simulink model "dc_motor_sim_model"  (R2017a)
settings: Solver=FixedStepAuto  StartTime=0.0  StopTime=0.5  FixedStep=1e-4  RelTol=1e-3
InitFcn:
  | Tw=0.01;     %Ancho de Ventana.
  | ppv=20;      %Pulsos por vuelta.
  | Ts=1e-4;     %Tiempo de muestreo.
  | 
  | num=[0 0.7770 0];
  | den=[1.0000 -0.9918 -0.0061];
settings Model: Creator=Martin  LastModifiedBy=Martin

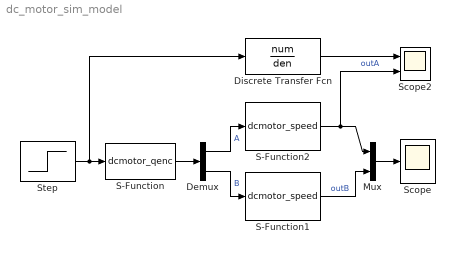
== system dc_motor_sim_model ==
  Demux : Demux  Outputs=2
  Discrete Transfer Fcn : DiscreteTransferFcn  Numerator=num  Denominator=den  SampleTime=Ts
  Mux : Mux  Inputs=2
  S-Function : S-Function  FunctionName=dcmotor_qenc  Parameters=ppv  SFunctionDeploymentMode=off  EnableBusSupport=off
  S-Function1 : S-Function  FunctionName=dcmotor_speed  Parameters=Ts,ppv,Tw  SFunctionDeploymentMode=off  EnableBusSupport=off
  S-Function2 : S-Function  FunctionName=dcmotor_speed  Parameters=Ts,ppv,Tw  SFunctionDeploymentMode=off  EnableBusSupport=off
  Scope : Scope
  Scope2 : Scope  NumInputPorts=2
  Step : Step  Time=0  After=12  SampleTime=Ts
  wires:
  S-Function/1 -> Demux/1
  Demux/2 -> S-Function1/1  "B"
  Demux/1 -> S-Function2/1  "A"
  Mux/1 -> Scope/1
  S-Function2/1 -> Mux/1, Scope2/2  "outA"
  S-Function1/1 -> Mux/2  "outB"
  Step/1 -> S-Function/1, Discrete Transfer Fcn/1
  Discrete Transfer Fcn/1 -> Scope2/1
